simulink model "task5_8"  (R2021a)
settings: Solver=VariableStepAuto  StartTime=0.0  StopTime=10.0  RelTol=1e-3
settings Model: Creator=reemb  LastModifiedBy=reemb

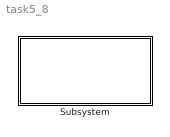
== system task5_8 ==
  Subsystem : Subsystem  mask{A=1, B=0}
      mask prompts: A "A VALUE"; B "B VALUE"

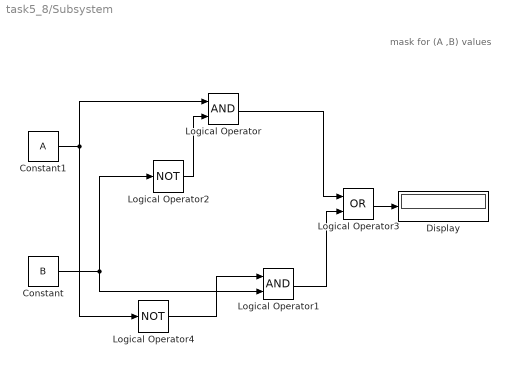
== system task5_8/Subsystem ==
  note: mask for (A ,B) values
  Constant : Constant  Value=B  OutDataTypeStr=boolean
  Constant1 : Constant  Value=A  OutDataTypeStr=boolean
  Display : Display
  Logical Operator : Logic  AllPortsSameDT=off  OutDataTypeStr=boolean
  Logical Operator1 : Logic  AllPortsSameDT=off  OutDataTypeStr=boolean
  Logical Operator2 : Logic  Operator=NOT  AllPortsSameDT=off  OutDataTypeStr=boolean
  Logical Operator3 : Logic  Operator=OR  AllPortsSameDT=off  OutDataTypeStr=boolean
  Logical Operator4 : Logic  Operator=NOT  AllPortsSameDT=off  OutDataTypeStr=boolean
  wires:
  Logical Operator1/1 -> Logical Operator3/2
  Constant1/1 -> Logical Operator4/1, Logical Operator/1
  Logical Operator2/1 -> Logical Operator/2
  Constant/1 -> Logical Operator2/1, Logical Operator1/2
  Logical Operator3/1 -> Display/1
  Logical Operator4/1 -> Logical Operator1/1
  Logical Operator/1 -> Logical Operator3/1
